simulink model "linear_h1"  (R2024b)
settings: Solver=VariableStepAuto  StartTime=0.0  StopTime=200.0  RelTol=1e-3
model workspace (MAT data in the model file):
  Cd = Simulink.Parameter
  Cd.Value = 0.3
  Cd.Complexity = 'real'
  Cd.Dimensions = [1 1]
  Cd.DataType = 'auto'
  D_1 = Simulink.Parameter
  D_1.Value = 0.045
  D_1.Complexity = 'real'
  D_1.Dimensions = [1 1]
  D_1.DataType = 'auto'
  D_o1 = Simulink.Parameter
  D_o1.Value = 0.005
  D_o1.Complexity = 'real'
  D_o1.Dimensions = [1 1]
  D_o1.DataType = 'auto'
  Kpump = 4e-06
  V_P0 = Simulink.Parameter
  V_P0.Value = 9
  V_P0.Complexity = 'real'
  V_P0.Dimensions = [1 1]
  V_P0.DataType = 'auto'
  g = Simulink.Parameter
  g.Value = 9.81
  g.Complexity = 'real'
  g.Dimensions = [1 1]
  g.DataType = 'auto'
  h_10 = Simulink.Parameter
  h_10.Value = 0.001
  h_10.Complexity = 'real'
  h_10.Dimensions = [1 1]
  h_10.DataType = 'auto'
settings Model: Creator=apm3  LastModifiedBy=baley

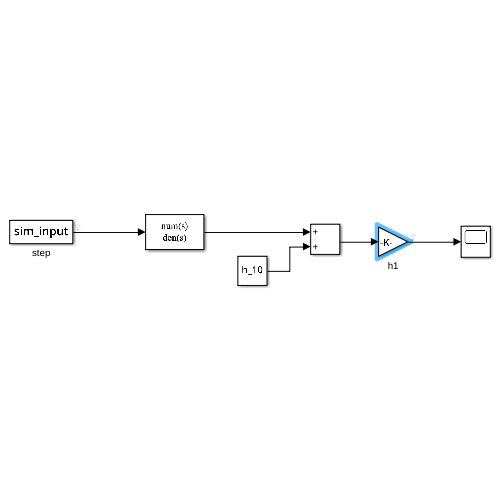
[thumbnail: Simulink's stored preview of the top-level diagram]
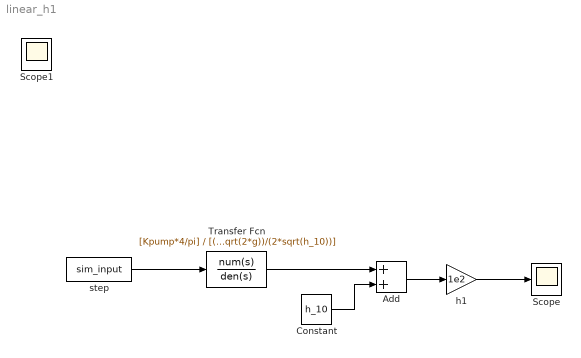
== system linear_h1 ==
  Add : Sum
  Constant : Constant  Value=h_10
  Scope : Scope
  Transfer Fcn : TransferFcn  Numerator=[Kpump*4/pi]  Denominator=[(D_1)^2 ((D_o1^2)*Cd*sqrt(2*g))/(2*sqrt(h_10))]
  h1 : Gain  Gain=1e2
  step : FromWorkspace  VariableName=sim_input
  Scope1 : Scope
  wires:
  step/1 -> Transfer Fcn/1
  Transfer Fcn/1 -> Add/1
  Constant/1 -> Add/2
  Add/1 -> h1/1
  h1/1 -> Scope/1
